simulink model "Furnance_Temperature_Control"  (R2025a)
settings: Solver=VariableStepAuto  StartTime=0.0  StopTime=50000  RelTol=1e-3
libraries: slpidlib x3, simulink x2
settings Model: NumberOfSteps=100  SnapshotBufferSize=100  SnapshotInterval=100  Creator=sarav  LastModifiedBy=sarav

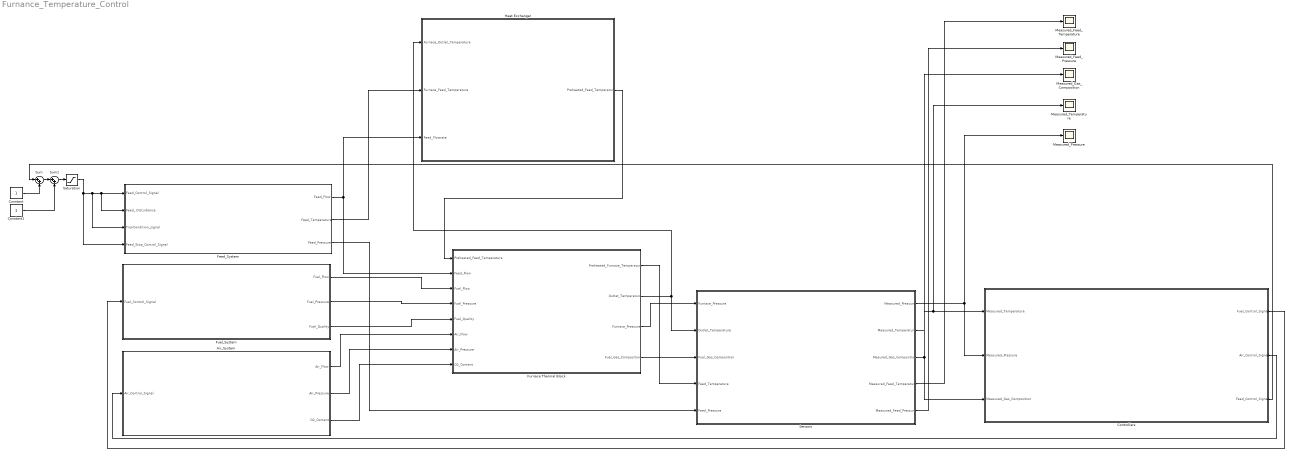
== system Furnance_Temperature_Control ==
  Air_System : Subsystem
  Constant : Constant
  Constant1 : Constant
  Controllers : Subsystem
  Feed_System : Subsystem
  Fuel_System : Subsystem
  Furnace Thermal Block : Subsystem
  Heat Exchanger : Subsystem
  Measured_Feed_Pressure : Scope
      settings: ActiveDisplayYMinimum=5.5036512639114221  ActiveDisplayYMaximum=6.42909560871398  DataLoggingVariableName=ScopeData2
  Measured_Feed_Temperature : Scope
      settings: ActiveDisplayYMinimum=81.966998560677908  ActiveDisplayYMaximum=82.009614071569516
  Measured_Gas_Composition : Scope
      settings: ActiveDisplayYMinimum=0.049999867381968433  ActiveDisplayYMaximum=0.050000059416157774  DataLoggingVariableName=ScopeData2
  Measured_Pressure : Scope
      settings: ActiveDisplayYMinimum=28.596753735230831  ActiveDisplayYMaximum=30.579970681505891
  Measured_Temperature : Scope
      settings: ActiveDisplayYMinimum=579.39513419742082  ActiveDisplayYMaximum=584.02036702549879
  Saturation : Saturate  UpperLimit=2  LowerLimit=0.5
  Sensors : Subsystem
  Sum : Sum  Inputs=|++  OutMin=1
  Sum1 : Sum  Inputs=|++
  wires:
  Fuel_System/1(Fuel_Flow) -> Furnace Thermal Block/3(Fuel_Flow)
  Feed_System/1(Feed_Flow) -> Heat Exchanger/3(Feed_Flowrate), Furnace Thermal Block/2(Feed_Flow)
  Air_System/1(Air_Flow) -> Furnace Thermal Block/6(Air_Flow)
  Furnace Thermal Block/3(Furnace_Pressure) -> Sensors/1(Furnace_Pressure)
  Sensors/2(Measured_Temperature) -> Measured_Temperature/1, Controllers/1(Measured_Temperature)
  Controllers/1(Fuel_Control_Signal) -> Fuel_System/1(Fuel_Control_Signal)
  Controllers/3(Feed_Control_Signal) -> Sum/1
  Controllers/2(Air_Control_Signal) -> Air_System/1(Air_Control_Signal)
  Constant/1 -> Sum/2
  Sum/1 -> Sum1/1
  Constant1/1 -> Sum1/2
  Feed_System/3(Feed_Pressure) -> Sensors/5(Feed_Pressure)
  Furnace Thermal Block/2(Outlet_Temperature) -> Sensors/2(Outlet_Temperature), Heat Exchanger/1(Furnace_Outlet_Temperature)
  Furnace Thermal Block/4(Fuel_Gas_Composition) -> Sensors/3(Fuel_Gas_Composition)
  Sensors/1(Measured_Pressure) -> Controllers/2(Measured_Pressure), Measured_Pressure/1
  Sensors/3(Meaured_Gas_Composition) -> Controllers/3(Measured_Gas_Composition), Measured_Gas_Composition/1
  Sensors/4(Measured_Feed_Temperature) -> Measured_Feed_Temperature/1
  Sensors/5(Measured_Feed_Pressure) -> Measured_Feed_Pressure/1
  Air_System/2(Air_Pressure) -> Furnace Thermal Block/7(Air_Pressure)
  Air_System/3(O2_Content) -> Furnace Thermal Block/8(O2_Content)
  Fuel_System/2(Fuel_Pressure) -> Furnace Thermal Block/4(Fuel_Pressure)
  Fuel_System/3(Fuel_Quality) -> Furnace Thermal Block/5(Fuel_Quality)
  Saturation/1 -> Feed_System/3(" Trip/Condition_signal"), Feed_System/1(Feed_Control_Signal), Feed_System/2(Feed_ Disturbance), Feed_System/4(Feed_Stop_Control_Signal)
  Sum1/1 -> Saturation/1
  Heat Exchanger/1(Preheated_Feed_Temperature) -> Furnace Thermal Block/1(Preheated_Feed_Temperature)
  Feed_System/2(Feed_Temperature) -> Heat Exchanger/2(Furnace_Feed_Temperature)
  Furnace Thermal Block/1(Preheated_Furnace_Temperature) -> Sensors/4(Feed_Temperature)

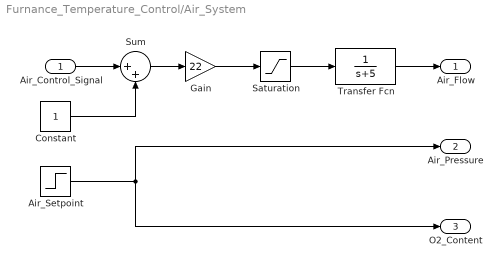
== system Furnance_Temperature_Control/Air_System ==
  Air_Control_Signal : Inport
  Air_Setpoint : Step  Time=50  Before=0.7  After=0.8  SampleTime=0
  Constant : Constant
  Gain : Gain  Gain=22
  Saturation : Saturate  UpperLimit=10001  LowerLimit=5000
  Sum : Sum  Inputs=|++
  Transfer Fcn : TransferFcn  Denominator=[1 5]
  Air_Flow : Outport
  Air_Pressure : Outport  Port=2
  O2_Content : Outport  Port=3
  wires:
  Air_Control_Signal/1 -> Sum/1
  Constant/1 -> Sum/2
  Sum/1 -> Gain/1
  Gain/1 -> Saturation/1
  Saturation/1 -> Transfer Fcn/1
  Transfer Fcn/1 -> Air_Flow/1
  Air_Setpoint/1 -> Air_Pressure/1, O2_Content/1

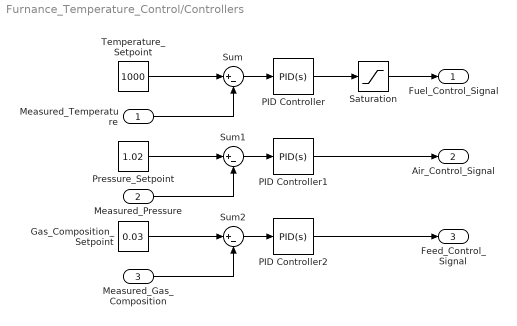
== system Furnance_Temperature_Control/Controllers ==
  Measured_Temperature : Inport
  Measured_Pressure : Inport  Port=2
  Measured_Gas_Composition : Inport  Port=3
  Gas_Composition_Setpoint : Constant  Value=0.03
  PID Controller : slpidlib/PID Controller  Controller=PID  Form=Parallel  TimeDomain=Continuous-time  UseExternalTs=off  SampleTime=-1  IntegratorMethod=Forward Euler  FilterMethod=Forward Euler  ControllerParametersSource=internal  P=0.1  I=0.01  UseKiTs=off  D=0  UseExternalDerivativeSource=off  N=100  UseFilter=on  TunerSelectOption=Transfer Function Based (PID Tuner App)  InitialConditionSource=internal  InitialConditionForIntegrator=0  InitialConditionForFilter=0  DifferentiatorICPrevScaledInput=0  ExternalReset=none  TrackingMode=off  Kt=1  LimitOutput=off  SatLimitsSource=internal  UpperSaturationLimit=inf  LowerSaturationLimit=-inf  LinearizeAsGain=on  AntiWindupMode=none  Kb=1  LimitIntegrator=off  UpperIntegratorSaturationLimit=inf  LowerIntegratorSaturationLimit=-inf  POutMin=[]  POutMax=[]  IOutMin=[]  IOutMax=[]  DOutMin=[]  DOutMax=[]  NOutMin=[]  NOutMax=[]  SumOutMin=[]  SumOutMax=[]  SaturationOutMin=[]  SaturationOutMax=[]  PParamMin=[]  PParamMax=[]  IParamMin=[]  IParamMax=[]  DParamMin=[]  DParamMax=[]  NParamMin=[]  NParamMax=[]  KbParamMin=[]  KbParamMax=[]  KtParamMin=[]  KtParamMax=[]  KbOutMin=[]  KbOutMax=[]  KtOutMin=[]  KtOutMax=[]  IntegratorOutMin=[]  IntegratorOutMax=[]  FilterOutMin=[]  FilterOutMax=[]  SumI1OutMin=[]  SumI1OutMax=[]  SumI2OutMin=[]  SumI2OutMax=[]  SumI3OutMin=[]  SumI3OutMax=[]  SumI4OutMin=[]  SumI4OutMax=[]  SumDOutMin=[]  SumDOutMax=[]  DifferentiatorOutMin=[]  DifferentiatorOutMax=[]  FilterDiffOutCoefMin=[]  FilterDiffOutCoefMax=[]  ReciprocalOutMin=[]  ReciprocalOutMax=[]  SumDenOutMin=[]  SumDenOutMax=[]  SumNumOutMin=[]  SumNumOutMax=[]  DivideOutMin=[]  DivideOutMax=[]  UdiffTsProdOutMin=[]  UdiffTsProdOutMax=[]  NTsProdOutMin=[]  NTsProdOutMax=[]  UintegralTsProdOutMin=[]  UintegralTsProdOutMax=[]  UngainTsProdOutMin=[]  UngainTsProdOutMax=[]  ClampingZeroOutDataTypeStr=Inherit: Inherit via back propagation  ClampingZeroOutMin=[]  ClampingZeroOutMax=[]  FilterDenConstantOutDataTypeStr=Inherit: Inherit via back propagation  FilterDenConstantOutMin=[]  FilterDenConstantOutMax=[]  PCopyOutDataTypeStr=Inherit: Inherit via back propagation  PCopyOutMin=[]  PCopyOutMax=[]  NCopyOutDataTypeStr=Inherit: Inherit via back propagation  NCopyOutMin=[]  NCopyOutMax=[]  IntegratorContinuousStateAttributes=''  IntegratorStateMustResolveToSignalObject=off  IntegratorRTWStateStorageClass=Auto  FilterContinuousStateAttributes=''  FilterStateMustResolveToSignalObject=off  FilterRTWStateStorageClass=Auto  ParallelPVariant=InternalParameters  IdealPVariant=Disabled  IVariant=InternalParameters  DVariant=InternalParameters  IntegratorVariant=Continuous  SatVariant=Disabled  AWVariant=Passthrough  PCopyVariant=Disabled  TRVariant=Disabled  FdbkBlocksVariant=Forward  IdealPFdbkVariant=Disabled  SatFdbkVariant=Disabled  DerivativeFilterVariant=ContFilter  NVariant=InternalParameters  NCopyVariant=Disabled  FilterICVariant=InternalICsFilter  IntegratorICVariant=InternalICs  ExternalResetVariant=Disabled  TRSumVariant=Passthrough  SumFdbkVariant=Disabled  SumVariant=Sum_PID  TsampFilterVariant=InternalTs  TsampNgainVariant=Passthrough  TsampIntegralVariant=Disabled_SignalSpec  ExternalSaturationOutDataTypeStr=Inherit: Same as second input  DerivativeSourceVariant=ErrorSignal  PreIntVariant=InternalPreInt
  PID Controller1 : slpidlib/PID Controller  Controller=PID  Form=Parallel  TimeDomain=Continuous-time  UseExternalTs=off  SampleTime=-1  IntegratorMethod=Forward Euler  FilterMethod=Forward Euler  ControllerParametersSource=internal  P=0.1  I=-0.01  UseKiTs=off  D=0  UseExternalDerivativeSource=off  N=100  UseFilter=on  TunerSelectOption=Transfer Function Based (PID Tuner App)  InitialConditionSource=internal  InitialConditionForIntegrator=0  InitialConditionForFilter=0  DifferentiatorICPrevScaledInput=0  ExternalReset=none  TrackingMode=off  Kt=1  LimitOutput=off  SatLimitsSource=internal  UpperSaturationLimit=inf  LowerSaturationLimit=-inf  LinearizeAsGain=on  AntiWindupMode=none  Kb=1  LimitIntegrator=off  UpperIntegratorSaturationLimit=inf  LowerIntegratorSaturationLimit=-inf  POutMin=[]  POutMax=[]  IOutMin=[]  IOutMax=[]  DOutMin=[]  DOutMax=[]  NOutMin=[]  NOutMax=[]  SumOutMin=[]  SumOutMax=[]  SaturationOutMin=[]  SaturationOutMax=[]  PParamMin=[]  PParamMax=[]  IParamMin=[]  IParamMax=[]  DParamMin=[]  DParamMax=[]  NParamMin=[]  NParamMax=[]  KbParamMin=[]  KbParamMax=[]  KtParamMin=[]  KtParamMax=[]  KbOutMin=[]  KbOutMax=[]  KtOutMin=[]  KtOutMax=[]  IntegratorOutMin=[]  IntegratorOutMax=[]  FilterOutMin=[]  FilterOutMax=[]  SumI1OutMin=[]  SumI1OutMax=[]  SumI2OutMin=[]  SumI2OutMax=[]  SumI3OutMin=[]  SumI3OutMax=[]  SumI4OutMin=[]  SumI4OutMax=[]  SumDOutMin=[]  SumDOutMax=[]  DifferentiatorOutMin=[]  DifferentiatorOutMax=[]  FilterDiffOutCoefMin=[]  FilterDiffOutCoefMax=[]  ReciprocalOutMin=[]  ReciprocalOutMax=[]  SumDenOutMin=[]  SumDenOutMax=[]  SumNumOutMin=[]  SumNumOutMax=[]  DivideOutMin=[]  DivideOutMax=[]  UdiffTsProdOutMin=[]  UdiffTsProdOutMax=[]  NTsProdOutMin=[]  NTsProdOutMax=[]  UintegralTsProdOutMin=[]  UintegralTsProdOutMax=[]  UngainTsProdOutMin=[]  UngainTsProdOutMax=[]  ClampingZeroOutDataTypeStr=Inherit: Inherit via back propagation  ClampingZeroOutMin=[]  ClampingZeroOutMax=[]  FilterDenConstantOutDataTypeStr=Inherit: Inherit via back propagation  FilterDenConstantOutMin=[]  FilterDenConstantOutMax=[]  PCopyOutDataTypeStr=Inherit: Inherit via back propagation  PCopyOutMin=[]  PCopyOutMax=[]  NCopyOutDataTypeStr=Inherit: Inherit via back propagation  NCopyOutMin=[]  NCopyOutMax=[]  IntegratorContinuousStateAttributes=''  IntegratorStateMustResolveToSignalObject=off  IntegratorRTWStateStorageClass=Auto  FilterContinuousStateAttributes=''  FilterStateMustResolveToSignalObject=off  FilterRTWStateStorageClass=Auto  ParallelPVariant=InternalParameters  IdealPVariant=Disabled  IVariant=InternalParameters  DVariant=InternalParameters  IntegratorVariant=Continuous  SatVariant=Disabled  AWVariant=Passthrough  PCopyVariant=Disabled  TRVariant=Disabled  FdbkBlocksVariant=Forward  IdealPFdbkVariant=Disabled  SatFdbkVariant=Disabled  DerivativeFilterVariant=ContFilter  NVariant=InternalParameters  NCopyVariant=Disabled  FilterICVariant=InternalICsFilter  IntegratorICVariant=InternalICs  ExternalResetVariant=Disabled  TRSumVariant=Passthrough  SumFdbkVariant=Disabled  SumVariant=Sum_PID  TsampFilterVariant=InternalTs  TsampNgainVariant=Passthrough  TsampIntegralVariant=Disabled_SignalSpec  ExternalSaturationOutDataTypeStr=Inherit: Same as second input  DerivativeSourceVariant=ErrorSignal  PreIntVariant=InternalPreInt
  PID Controller2 : slpidlib/PID Controller  Controller=PID  Form=Parallel  TimeDomain=Continuous-time  UseExternalTs=off  SampleTime=-1  IntegratorMethod=Forward Euler  FilterMethod=Forward Euler  ControllerParametersSource=internal  P=0.1  I=0.01  UseKiTs=off  D=0  UseExternalDerivativeSource=off  N=100  UseFilter=on  TunerSelectOption=Transfer Function Based (PID Tuner App)  InitialConditionSource=internal  InitialConditionForIntegrator=0  InitialConditionForFilter=0  DifferentiatorICPrevScaledInput=0  ExternalReset=none  TrackingMode=off  Kt=1  LimitOutput=off  SatLimitsSource=internal  UpperSaturationLimit=inf  LowerSaturationLimit=-inf  LinearizeAsGain=on  AntiWindupMode=none  Kb=1  LimitIntegrator=off  UpperIntegratorSaturationLimit=inf  LowerIntegratorSaturationLimit=-inf  POutMin=[]  POutMax=[]  IOutMin=[]  IOutMax=[]  DOutMin=[]  DOutMax=[]  NOutMin=[]  NOutMax=[]  SumOutMin=[]  SumOutMax=[]  SaturationOutMin=[]  SaturationOutMax=[]  PParamMin=[]  PParamMax=[]  IParamMin=[]  IParamMax=[]  DParamMin=[]  DParamMax=[]  NParamMin=[]  NParamMax=[]  KbParamMin=[]  KbParamMax=[]  KtParamMin=[]  KtParamMax=[]  KbOutMin=[]  KbOutMax=[]  KtOutMin=[]  KtOutMax=[]  IntegratorOutMin=[]  IntegratorOutMax=[]  FilterOutMin=[]  FilterOutMax=[]  SumI1OutMin=[]  SumI1OutMax=[]  SumI2OutMin=[]  SumI2OutMax=[]  SumI3OutMin=[]  SumI3OutMax=[]  SumI4OutMin=[]  SumI4OutMax=[]  SumDOutMin=[]  SumDOutMax=[]  DifferentiatorOutMin=[]  DifferentiatorOutMax=[]  FilterDiffOutCoefMin=[]  FilterDiffOutCoefMax=[]  ReciprocalOutMin=[]  ReciprocalOutMax=[]  SumDenOutMin=[]  SumDenOutMax=[]  SumNumOutMin=[]  SumNumOutMax=[]  DivideOutMin=[]  DivideOutMax=[]  UdiffTsProdOutMin=[]  UdiffTsProdOutMax=[]  NTsProdOutMin=[]  NTsProdOutMax=[]  UintegralTsProdOutMin=[]  UintegralTsProdOutMax=[]  UngainTsProdOutMin=[]  UngainTsProdOutMax=[]  ClampingZeroOutDataTypeStr=Inherit: Inherit via back propagation  ClampingZeroOutMin=[]  ClampingZeroOutMax=[]  FilterDenConstantOutDataTypeStr=Inherit: Inherit via back propagation  FilterDenConstantOutMin=[]  FilterDenConstantOutMax=[]  PCopyOutDataTypeStr=Inherit: Inherit via back propagation  PCopyOutMin=[]  PCopyOutMax=[]  NCopyOutDataTypeStr=Inherit: Inherit via back propagation  NCopyOutMin=[]  NCopyOutMax=[]  IntegratorContinuousStateAttributes=''  IntegratorStateMustResolveToSignalObject=off  IntegratorRTWStateStorageClass=Auto  FilterContinuousStateAttributes=''  FilterStateMustResolveToSignalObject=off  FilterRTWStateStorageClass=Auto  ParallelPVariant=InternalParameters  IdealPVariant=Disabled  IVariant=InternalParameters  DVariant=InternalParameters  IntegratorVariant=Continuous  SatVariant=Disabled  AWVariant=Passthrough  PCopyVariant=Disabled  TRVariant=Disabled  FdbkBlocksVariant=Forward  IdealPFdbkVariant=Disabled  SatFdbkVariant=Disabled  DerivativeFilterVariant=ContFilter  NVariant=InternalParameters  NCopyVariant=Disabled  FilterICVariant=InternalICsFilter  IntegratorICVariant=InternalICs  ExternalResetVariant=Disabled  TRSumVariant=Passthrough  SumFdbkVariant=Disabled  SumVariant=Sum_PID  TsampFilterVariant=InternalTs  TsampNgainVariant=Passthrough  TsampIntegralVariant=Disabled_SignalSpec  ExternalSaturationOutDataTypeStr=Inherit: Same as second input  DerivativeSourceVariant=ErrorSignal  PreIntVariant=InternalPreInt
  Pressure_Setpoint : Constant  Value=1.02
  Saturation : Saturate  UpperLimit=6000  LowerLimit=1500
  Sum : Sum  Inputs=|+-
  Sum1 : Sum  Inputs=|+-
  Sum2 : Sum  Inputs=|+-
  Temperature_Setpoint : Constant  Value=1000
  Fuel_Control_Signal : Outport
  Air_Control_Signal : Outport  Port=2
  Feed_Control_Signal : Outport  Port=3
  wires:
  Temperature_Setpoint/1 -> Sum/1
  Measured_Temperature/1 -> Sum/2
  Sum/1 -> PID Controller/1
  PID Controller/1 -> Saturation/1
  Pressure_Setpoint/1 -> Sum1/1
  Measured_Pressure/1 -> Sum1/2
  Sum1/1 -> PID Controller1/1
  PID Controller1/1 -> Air_Control_Signal/1
  Gas_Composition_Setpoint/1 -> Sum2/1
  Measured_Gas_Composition/1 -> Sum2/2
  Sum2/1 -> PID Controller2/1
  PID Controller2/1 -> Feed_Control_Signal/1
  Saturation/1 -> Fuel_Control_Signal/1

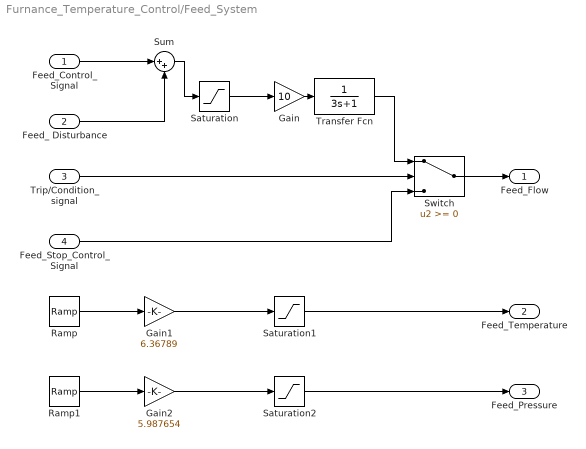
== system Furnance_Temperature_Control/Feed_System ==
  Feed_Control_Signal : Inport  OutMin=0.1  OutMax=10  SampleTime=1  LockScale=on
  Feed_ Disturbance : Inport  Port=2  OutMin=0.1  OutMax=10  SampleTime=1
  " Trip/Condition_signal" : Inport  Port=3  OutMin=0  OutMax=10  LockScale=on
  Feed_Stop_Control_Signal : Inport  Port=4  OutMin=10  OutMax=20  LockScale=on
  Gain : Gain  Gain=10
  Gain1 : Gain  Gain=6.36789
  Gain2 : Gain  Gain=5.987654
  Ramp : simulink/Sources/Ramp  slope=1  start=0  InitialOutput=7
  Ramp1 : simulink/Sources/Ramp  slope=0.005  start=0  InitialOutput=0.2
  Saturation : Saturate  UpperLimit=585  LowerLimit=4.68934985
  Saturation1 : Saturate  UpperLimit=80.001  LowerLimit=0
  Saturation2 : Saturate  UpperLimit=6  LowerLimit=3
  Sum : Sum  Inputs=|++
  Switch : Switch  SaturateOnIntegerOverflow=off  InputSameDT=off
  Transfer Fcn : TransferFcn  Denominator=[3 1]
  Feed_Flow : Outport  OutMin=100000  OutMax=100000
  Feed_Temperature : Outport  Port=2
  Feed_Pressure : Outport  Port=3
  wires:
  Feed_Control_Signal/1 -> Sum/1
  Feed_ Disturbance/1 -> Sum/2
  Sum/1 -> Saturation/1
  Ramp/1 -> Gain1/1
  Ramp1/1 -> Gain2/1
  Saturation/1 -> Gain/1
  Gain/1 -> Transfer Fcn/1
  Feed_Stop_Control_Signal/1 -> Switch/3
  " Trip/Condition_signal"/1 -> Switch/2
  Transfer Fcn/1 -> Switch/1
  Switch/1 -> Feed_Flow/1
  Gain1/1 -> Saturation1/1
  Saturation1/1 -> Feed_Temperature/1
  Gain2/1 -> Saturation2/1
  Saturation2/1 -> Feed_Pressure/1

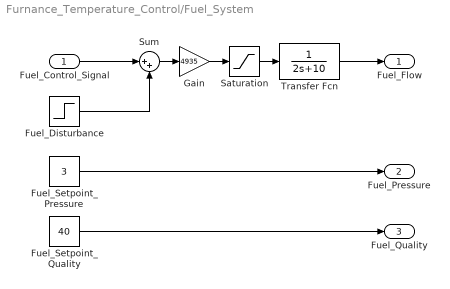
== system Furnance_Temperature_Control/Fuel_System ==
  Fuel_Control_Signal : Inport
  Fuel_Disturbance : Step  Time=50  After=-0.1  SampleTime=0
  Fuel_Setpoint_Pressure : Constant  Value=3
  Fuel_Setpoint_Quality : Constant  Value=40
  Gain : Gain  Gain=4935
  Saturation : Saturate  UpperLimit=10000  LowerLimit=5000
  Sum : Sum  Inputs=|++
  Transfer Fcn : TransferFcn  Denominator=[2 10]
  Fuel_Flow : Outport
  Fuel_Pressure : Outport  Port=2
  Fuel_Quality : Outport  Port=3
  wires:
  Fuel_Control_Signal/1 -> Sum/1
  Fuel_Disturbance/1 -> Sum/2
  Sum/1 -> Gain/1
  Gain/1 -> Saturation/1
  Saturation/1 -> Transfer Fcn/1
  Transfer Fcn/1 -> Fuel_Flow/1
  Fuel_Setpoint_Pressure/1 -> Fuel_Pressure/1
  Fuel_Setpoint_Quality/1 -> Fuel_Quality/1

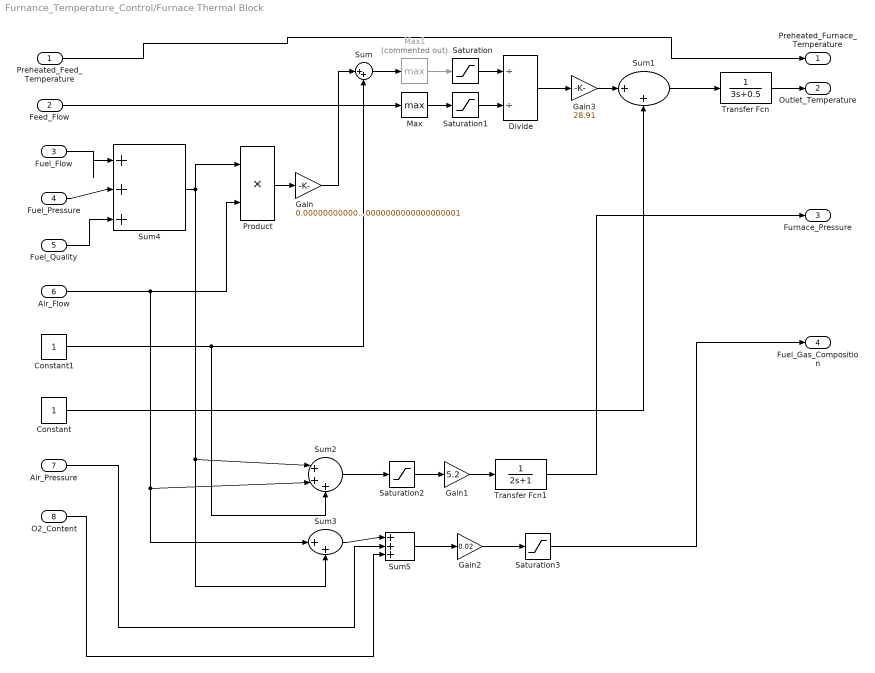
== system Furnance_Temperature_Control/Furnace Thermal Block ==
  Preheated_Feed_Temperature : Inport
  Feed_Flow : Inport  Port=2
  Fuel_Flow : Inport  Port=3
  Fuel_Pressure : Inport  Port=4
  Fuel_Quality : Inport  Port=5
  Air_Flow : Inport  Port=6  OutMin=0.1  OutMax=2
  Air_Pressure : Inport  Port=7
  O2_Content : Inport  Port=8
  Constant : Constant
  Constant1 : Constant
  Divide : Product  Inputs=//
  Gain : Gain  Gain=0.00000000000000000000000000000000000000000001
  Gain1 : Gain  Gain=5.2
  Gain2 : Gain  Gain=0.02
  Gain3 : Gain  Gain=28.91
  Max : MinMax  Function=max
  Max1 : MinMax  Commented=on  Function=max  InputSameDT=on
  Product : Product
  Saturation : Saturate  UpperLimit=10  LowerLimit=0.01
  Saturation1 : Saturate  UpperLimit=10  LowerLimit=0.01
  Saturation2 : Saturate  UpperLimit=0.2689  LowerLimit=0.00001
  Saturation3 : Saturate  UpperLimit=0.05  LowerLimit=0
  Sum : Sum  Inputs=|++
  Sum1 : Sum  Inputs=|++
  Sum2 : Sum  Inputs=|+++
  Sum3 : Sum  Inputs=|++
  Sum4 : Sum  Inputs=|+++
  Sum5 : Sum  Inputs=|+++
  Transfer Fcn : TransferFcn  Denominator=[3 0.5]  ParameterTunability=Optimized
  Transfer Fcn1 : TransferFcn  Denominator=[2 1]
  Preheated_Furnace_Temperature : Outport
  Outlet_Temperature : Outport  Port=2
  Furnace_Pressure : Outport  Port=3
  Fuel_Gas_Composition : Outport  Port=4
  wires:
  Sum4/1 -> Sum3/2, Sum2/1, Product/1
  Air_Flow/1 -> Sum2/2, Sum3/1, Product/2
  Product/1 -> Gain/1
  Gain/1 -> Sum/1
  Constant1/1 -> Sum2/3, Sum/2
  Sum/1 -> Max1/1
  Feed_Flow/1 -> Max/1
  Constant/1 -> Sum1/2
  Sum2/1 -> Saturation2/1
  Gain1/1 -> Transfer Fcn1/1
  Sum3/1 -> Sum5/1
  Gain2/1 -> Saturation3/1
  Max1/1 -> Saturation/1
  Max/1 -> Saturation1/1
  Saturation/1 -> Divide/1
  Saturation1/1 -> Divide/2
  Transfer Fcn/1 -> Outlet_Temperature/1
  Sum1/1 -> Transfer Fcn/1
  Gain3/1 -> Sum1/1
  Divide/1 -> Gain3/1
  Saturation2/1 -> Gain1/1
  Transfer Fcn1/1 -> Furnace_Pressure/1
  Saturation3/1 -> Fuel_Gas_Composition/1
  Fuel_Flow/1 -> Sum4/1
  Fuel_Pressure/1 -> Sum4/2
  Fuel_Quality/1 -> Sum4/3
  Air_Pressure/1 -> Sum5/2
  O2_Content/1 -> Sum5/3
  Sum5/1 -> Gain2/1
  Preheated_Feed_Temperature/1 -> Preheated_Furnace_Temperature/1

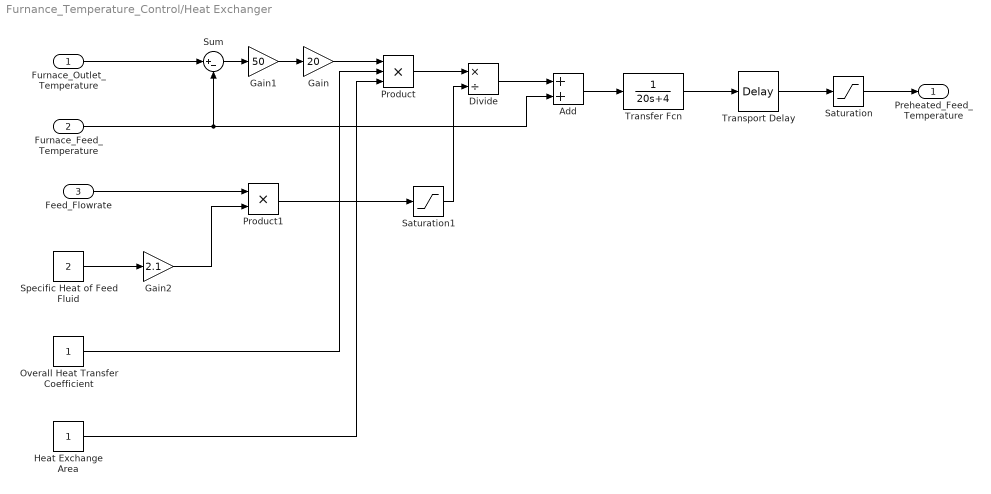
== system Furnance_Temperature_Control/Heat Exchanger ==
  Furnace_Outlet_Temperature : Inport
  Furnace_Feed_Temperature : Inport  Port=2
  Feed_Flowrate : Inport  Port=3
  Add : Sum
  Divide : Product  Inputs=*/
  Gain : Gain  Gain=20
  Gain1 : Gain  Gain=50
  Gain2 : Gain  Gain=2.1
  Heat Exchange Area : Constant
  Overall Heat Transfer Coefficient : Constant
  Product : Product  Inputs=3
  Product1 : Product
  Saturation : Saturate  UpperLimit=160  LowerLimit=80
  Saturation1 : Saturate  UpperLimit=10  LowerLimit=0.5
  Specific Heat of Feed Fluid : Constant  Value=2
  Sum : Sum  Inputs=|+-
  Transfer Fcn : TransferFcn  Denominator=[20 4]
  Transport Delay : TransportDelay  DelayTime=05  InitialOutput=81  FixedBuffer=on  TransDelayFeedthrough=on  PadeOrder=50
  Preheated_Feed_Temperature : Outport
  wires:
  Furnace_Outlet_Temperature/1 -> Sum/1
  Furnace_Feed_Temperature/1 -> Add/2, Sum/2
  Sum/1 -> Gain1/1
  Overall Heat Transfer Coefficient/1 -> Product/2
  Heat Exchange Area/1 -> Product/3
  Feed_Flowrate/1 -> Product1/1
  Specific Heat of Feed Fluid/1 -> Gain2/1
  Product1/1 -> Saturation1/1
  Product/1 -> Divide/1
  Divide/1 -> Add/1
  Gain1/1 -> Gain/1
  Transport Delay/1 -> Saturation/1
  Saturation/1 -> Preheated_Feed_Temperature/1
  Gain/1 -> Product/1
  Gain2/1 -> Product1/2
  Add/1 -> Transfer Fcn/1
  Saturation1/1 -> Divide/2
  Transfer Fcn/1 -> Transport Delay/1

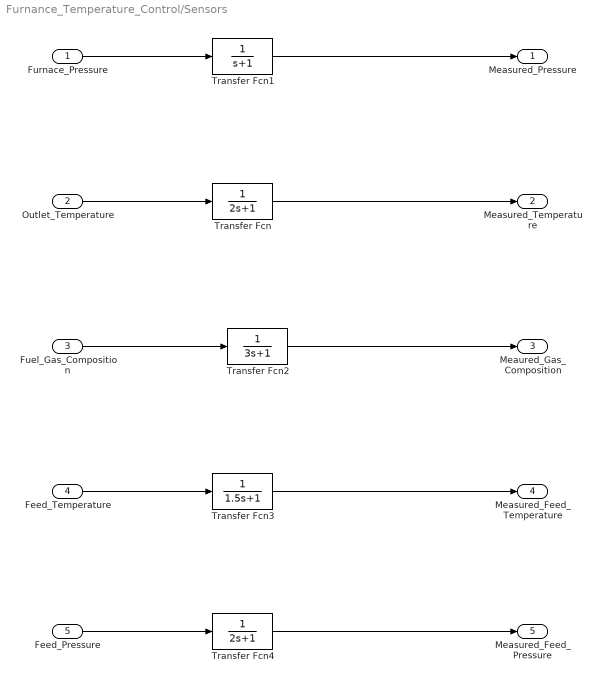
== system Furnance_Temperature_Control/Sensors ==
  Furnace_Pressure : Inport
  Outlet_Temperature : Inport  Port=2
  Fuel_Gas_Composition : Inport  Port=3
  Feed_Temperature : Inport  Port=4
  Feed_Pressure : Inport  Port=5
  Transfer Fcn : TransferFcn  Denominator=[2 1]
  Transfer Fcn1 : TransferFcn  Denominator=[1 1]
  Transfer Fcn2 : TransferFcn  Denominator=[3 1]
  Transfer Fcn3 : TransferFcn  Denominator=[1.5 1]
  Transfer Fcn4 : TransferFcn  Denominator=[2 1]
  Measured_Pressure : Outport
  Measured_Temperature : Outport  Port=2
  Meaured_Gas_Composition : Outport  Port=3
  Measured_Feed_Temperature : Outport  Port=4
  Measured_Feed_Pressure : Outport  Port=5
  wires:
  Outlet_Temperature/1 -> Transfer Fcn/1
  Transfer Fcn/1 -> Measured_Temperature/1
  Furnace_Pressure/1 -> Transfer Fcn1/1
  Transfer Fcn1/1 -> Measured_Pressure/1
  Feed_Temperature/1 -> Transfer Fcn3/1
  Transfer Fcn3/1 -> Measured_Feed_Temperature/1
  Feed_Pressure/1 -> Transfer Fcn4/1
  Transfer Fcn4/1 -> Measured_Feed_Pressure/1
  Fuel_Gas_Composition/1 -> Transfer Fcn2/1
  Transfer Fcn2/1 -> Meaured_Gas_Composition/1
